simulink model "Series_Dynamic"  (R2015b)
settings: Solver=VariableStepAuto  StartTime=0.0  StopTime=20  RelTol=1e-3
undefined symbols (not defined in the file): A, C, f, g, gear, M, motors, p, r, Vw
settings Model: Creator=ihong-gyu  LastModifiedBy=ihong-gyu

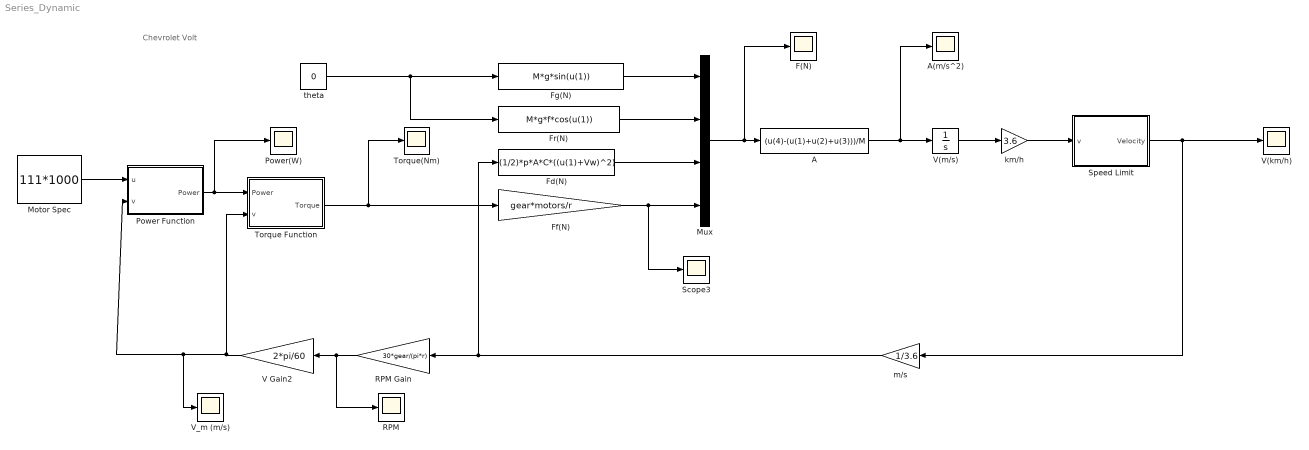
== system Series_Dynamic ==
  note: Chevrolet Volt
  A : Fcn  Expr=(u(4)-(u(1)+u(2)+u(3)))/M
  A(m/s^2) : Scope
  F(N) : Scope
  Fd(N) : Fcn  Expr=(1/2)*p*A*C*((u(1)+Vw)^2)
  Ff(N) : Gain  Gain=gear*motors/r
  Fg(N) : Fcn  Expr=M*g*sin(u(1))
  Fr(N) : Fcn  Expr=M*g*f*cos(u(1))
  Motor Spec : Constant  Value=111*1000
  Mux : Mux
  Power Function : MATLAB Function  TreatAsAtomicUnit=on
  Power(W) : Scope
  RPM : Scope
  RPM Gain : Gain  Gain=30*gear/(pi*r)
  Scope3 : Scope
  Speed Limit : MATLAB Function  TreatAsAtomicUnit=on
  "Torque Function " : MATLAB Function  TreatAsAtomicUnit=on
  Torque(Nm) : Scope
  V Gain2 : Gain  Gain=2*pi/60
  V(km/h) : Scope
  V(m/s) : Integrator
  V_m (m/s) : Scope
  km/h : Gain  Gain=3.6
  m/s : Gain  Gain=1/3.6
  theta : Constant  Value=0
  wires:
  Motor Spec/1 -> Power Function/1(u)
  Power Function/1(Power) -> Power(W)/1, "Torque Function "/1(Power)
  Fg(N)/1 -> Mux/1
  Fr(N)/1 -> Mux/2
  Fd(N)/1 -> Mux/3
  Mux/1 -> F(N)/1, A/1
  theta/1 -> Fr(N)/1, Fg(N)/1
  "Torque Function "/1(Torque) -> Torque(Nm)/1, Ff(N)/1
  A/1 -> V(m/s)/1, A(m/s^2)/1
  RPM Gain/1 -> RPM/1, V Gain2/1
  Ff(N)/1 -> Scope3/1, Mux/4
  V Gain2/1 -> "Torque Function "/2(v), V_m (m/s)/1, Power Function/2(v)
  km/h/1 -> Speed Limit/1(v)
  Speed Limit/1(Velocity) -> m/s/1, V(km/h)/1
  V(m/s)/1 -> km/h/1
  m/s/1 -> Fd(N)/1, RPM Gain/1

== matlab function Series_Dynamic/Torque Function  ==
  data: Power input; v input; Torque output
function Torque = fcn(Power, v)
%#codegen

if(Power~=111*1000)
    Torque = 398;
else
    Torque = Power/v;
end

== matlab function Series_Dynamic/Power Function ==
  data: u input; Power output; v input
function Power = fcn(u, v)
%#codegen

if(v~=0)
    Power=v*398;
else
    Power=1;
end

if(Power>111*1000)
    Power=111*1000;
end

== matlab function Series_Dynamic/Speed Limit ==
  data: v input; Velocity output
function Velocity = fcn(v)
%#codegen

if(v>154)
    Velocity=154;
else
    Velocity=v;
end
